simulink model "v1_lqi_observer"  (R2023b)
settings: Solver=VariableStepAuto  StartTime=0.0  StopTime=20  RelTol=1e-10
values from neighbouring files (symbols this model uses):
  A = [-p1-x_eq(2) -x_eq(1); 0 -p2]    [WP3.m]
  B = [0; p3]    [WP3.m]
  C = [1 0]    [WP3.m]
  K = [-49.7747 99.1105]    [WP3.m]
  L = eval(L)    [WP3.m]
  u_eq = 1.003    [WP3.m]
  x1_eq = x_eq(1)    [WP3.m]
  x_eq = [0.0451; 0.3099]    [WP3.m]
settings Model: Creator=kiraa  LastModifiedBy=david

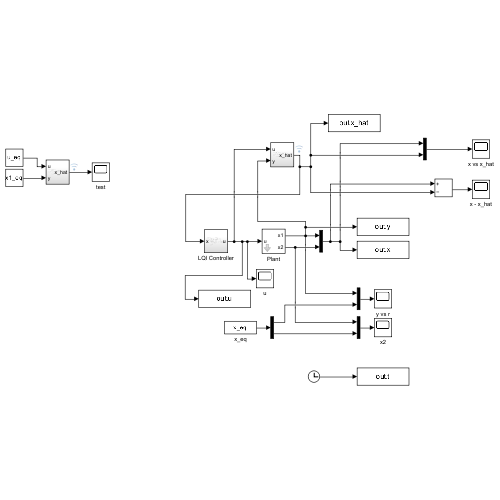
[thumbnail: Simulink's stored preview of the top-level diagram]
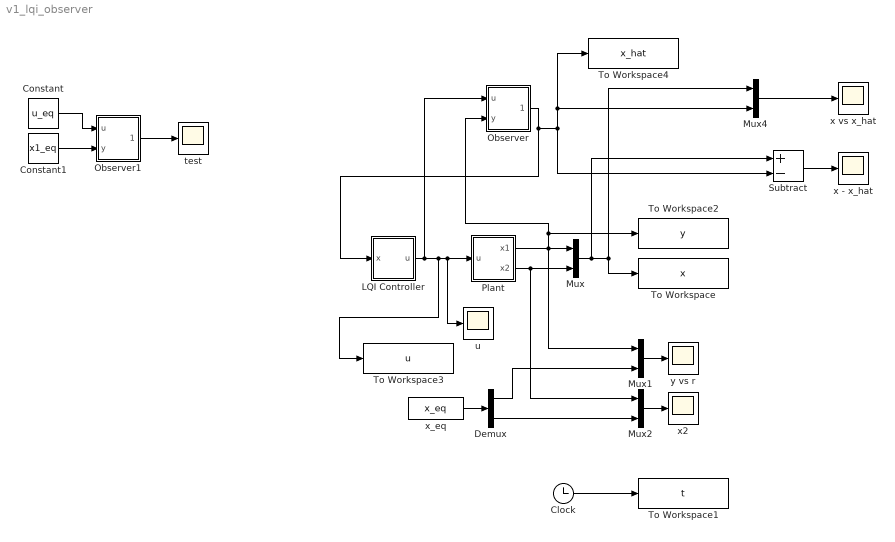
== system v1_lqi_observer ==
  Clock : Clock
  Constant : Constant  Value=u_eq
  Constant1 : Constant  Value=x1_eq
  Demux : Demux  Outputs=2
  LQI Controller : Subsystem
  Mux{,1..2,4} (4 alike) : Mux  Inputs=2
  Observer : Subsystem
  Observer1 : Subsystem
  Plant : Subsystem  mask{x1_0=0.1, x2_0=0}
      mask prompts: x1_0 "x1(0) [g/l]"; x2_0 "x2(0) [min^-1]"
  Subtract : Sum  Inputs=+-
  To Workspace : ToWorkspace  VariableName=x  SampleTime=-1
  To Workspace1 : ToWorkspace  VariableName=t  SaveFormat=Timeseries  SampleTime=-1
  To Workspace2 : ToWorkspace  VariableName=y  SampleTime=-1
  To Workspace3 : ToWorkspace  VariableName=u  SampleTime=-1
  To Workspace4 : ToWorkspace  VariableName=x_hat  SaveFormat=Timeseries  SampleTime=-1
  test : Scope
  u : Scope
  x - x_hat : Scope
  x vs x_hat : Scope
  x2 : Scope
  x_eq : Constant  Value=x_eq
  y vs r : Scope
  wires:
  Plant/2(x2) -> Mux2/1, Mux/2
  Mux/1 -> Subtract/1, Mux4/1, To Workspace/1
  Mux1/1 -> y vs r/1
  Demux/1 -> Mux1/2
  x_eq/1 -> Demux/1
  Demux/2 -> Mux2/2
  Mux2/1 -> x2/1
  Clock/1 -> To Workspace1/1
  LQI Controller/1(u) -> Observer/1(u), To Workspace3/1, Plant/1(u), u/1
  Plant/1(x1) -> Mux/1, Observer/2(y), To Workspace2/1, Mux1/1
  Mux4/1 -> x vs x_hat/1
  Observer/1(x_hat) -> LQI Controller/1(x), To Workspace4/1, Mux4/2, Subtract/2
  Subtract/1 -> x - x_hat/1
  Constant/1 -> Observer1/1(u)
  Constant1/1 -> Observer1/2(y)
  Observer1/1(x_hat) -> test/1

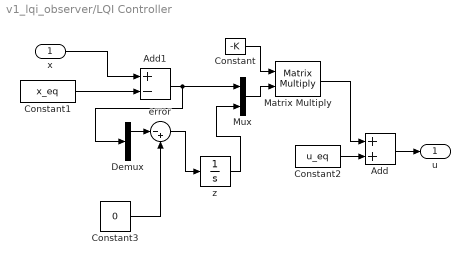
== system v1_lqi_observer/LQI Controller ==
  x : Inport
  Add : Sum
  Add1 : Sum  Inputs=+-  InputSameDT=on  LockScale=on
  Constant : Constant  Value=-K  VectorParams1D=off
  Constant1 : Constant  Value=x_eq
  Constant2 : Constant  Value=u_eq
  Constant3 : Constant  Value=0
  Demux : Demux  Outputs=2
  Matrix Multiply : Product  Multiplication=Matrix(*)
  Mux : Mux  Inputs=2
  error : Sum  Inputs=|-+
  z : Integrator  InitialCondition=0.1
  u : Outport
  wires:
  Constant/1 -> Matrix Multiply/1
  Matrix Multiply/1 -> Add/1
  Add/1 -> u/1
  Constant2/1 -> Add/2
  Constant1/1 -> Add1/2
  x/1 -> Add1/1
  Add1/1 -> Demux/1, Mux/1
  Mux/1 -> Matrix Multiply/2
  z/1 -> Mux/2
  Demux/1 -> error/1
  error/1 -> z/1
  Constant3/1 -> error/2

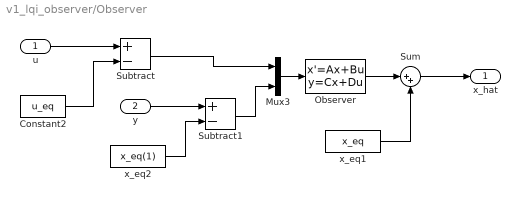
== system v1_lqi_observer/Observer ==
  u : Inport
  y : Inport  Port=2
  Constant2 : Constant  Value=u_eq
  Mux3 : Mux  Inputs=2
  Observer : StateSpace  A=A-L*C  B=[B L]  C=eye(2)  D=[0 0; 0 0]  InitialCondition=[0 0]  ParameterTunability=Unconstrained
  Subtract : Sum  Inputs=+-
  Subtract1 : Sum  Inputs=+-
  Sum : Sum  Inputs=|++
  x_eq1 : Constant  Value=x_eq
  x_eq2 : Constant  Value=x_eq(1)
  x_hat : Outport
  wires:
  u/1 -> Subtract/1
  Subtract1/1 -> Mux3/2
  Subtract/1 -> Mux3/1
  x_eq2/1 -> Subtract1/2
  x_eq1/1 -> Sum/2
  Mux3/1 -> Observer/1
  Constant2/1 -> Subtract/2
  Observer/1 -> Sum/1
  Sum/1 -> x_hat/1
  y/1 -> Subtract1/1

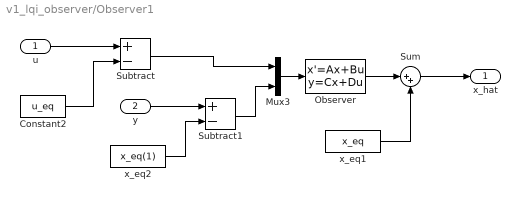
== system v1_lqi_observer/Observer1 ==
  u : Inport
  y : Inport  Port=2
  Constant2 : Constant  Value=u_eq
  Mux3 : Mux  Inputs=2
  Observer : StateSpace  A=A-L*C  B=[B L]  C=eye(2)  D=[0 0; 0 0]  InitialCondition=[0.001 0.01]  ParameterTunability=Unconstrained
  Subtract : Sum  Inputs=+-
  Subtract1 : Sum  Inputs=+-
  Sum : Sum  Inputs=|++
  x_eq1 : Constant  Value=x_eq
  x_eq2 : Constant  Value=x_eq(1)
  x_hat : Outport
  wires:
  u/1 -> Subtract/1
  Subtract1/1 -> Mux3/2
  Subtract/1 -> Mux3/1
  x_eq2/1 -> Subtract1/2
  x_eq1/1 -> Sum/2
  Mux3/1 -> Observer/1
  Constant2/1 -> Subtract/2
  Observer/1 -> Sum/1
  Sum/1 -> x_hat/1
  y/1 -> Subtract1/1

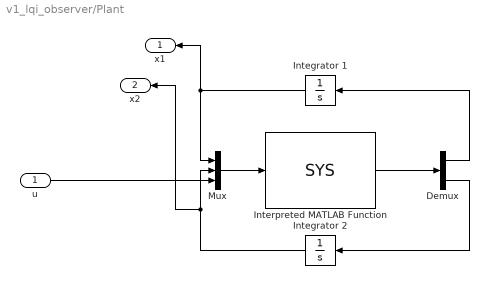
== system v1_lqi_observer/Plant ==
  u : Inport
  Demux : Demux  Outputs=2
  Integrator 1 : Integrator  InitialCondition=x1_0
  Integrator 2 : Integrator  InitialCondition=x2_0
  Interpreted MATLAB Function : MATLABFcn  MATLABFcn=SYS  OutputDimensions=2
  Mux : Mux  Inputs=3
  x1 : Outport
  x2 : Outport  Port=2
  wires:
  Integrator 1/1 -> x1/1, Mux/1
  Demux/1 -> Integrator 1/1
  Mux/1 -> Interpreted MATLAB Function/1
  Integrator 2/1 -> x2/1, Mux/2
  Interpreted MATLAB Function/1 -> Demux/1
  Demux/2 -> Integrator 2/1
  u/1 -> Mux/3
